simulink model "s_hover_lqrV2"  (R2012b)
settings: Solver=ode45  StartTime=0.0  StopTime=inf  FixedStep=0.01  RelTol=1e-3
values from neighbouring files (symbols this model uses):
  A = 6*(f2-f3)/z3+3*(d2+d3)    [LQRDiscretoFUNC.m]
  B = 3*(f3-f2)-z3*(d3+2*d2)    [LQRDiscretoFUNC.m]
  K = reshape(K, 4 , 6)    [LQRDiscretoFUNC.m]
undefined symbols (not defined in the file or in its folder): C, CMD_RATE_LIMIT, D, K_AMP, LQRDiscretoFUNC, V_bias, VMAX_AMP, VMAX_DAC, wcf, zetaf
libraries: simulink_extras x5, rtwinlib x1
settings Model: ExtModeTrigDuration=10000  Creator=hpineros  LastModifiedBy=David
settings SolverCC: PositivePriorityOrder=on
settings DataIOCC: SignalLoggingSaveFormat=ModelDataLogs
settings OptimizationCC: InitFltsAndDblsToZero=on
settings DebuggingCC: SaveWithParameterizedLinksMsg=none  FcnCallInpInsideContextMsg=UseLocalSettings  StrictBusMsg=Warning
settings RTWCC: SystemTargetFile=quarc_windows.tlc  TemplateMakefile=quarc_default_tmf  Description=QuaRC Win32 Target  ProcessScript=quarc_windows_make_rtw_hook
settings STFCustomTargetCC: TargetFcnLib=ansi_tfl_tmw.mat  TargetPreCompLibLocation=C:\DOCUME~1\ALLUSE~1\APPLIC~1\QUARC\lib\2007a\windows\release  CodeReplacementLibrary=ANSI_C  GeneratePreprocessorConditionals=Disable all  SystemTargetFile=quarc_windows.tlc
settings GRTTargetCC: TargetFcnLib=ansi_tfl_tmw.mat  TargetPreCompLibLocation=C:\DOCUME~1\ALLUSE~1\APPLIC~1\QUARC\lib\2007a\windows\release  ParMdlRefBuildCompliant=off  CompOptLevelCompliant=off  ConcurrentExecutionCompliant=off  CombineOutputUpdateFcns=off  MatFileLogging=off  GRTInterface=on  ExtMode=on  ExtModeMexFile=quarc_comm

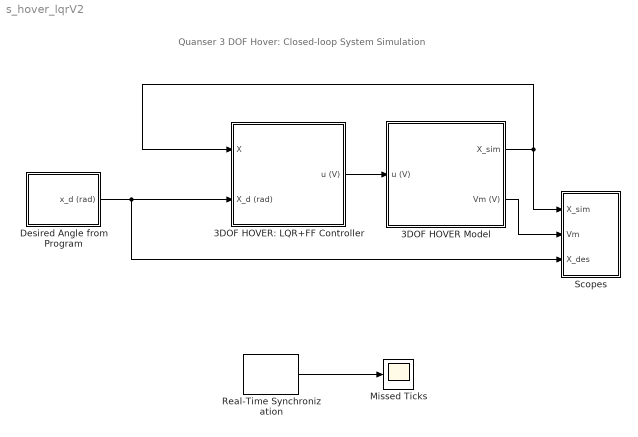
== system s_hover_lqrV2 ==
  note: Quanser 3 DOF Hover:
      | Closed-loop System Simulation
  3DOF HOVER Model : Subsystem
  3DOF HOVER: LQR+FF Controller : Subsystem
  Desired Angle from Program : Subsystem
  Missed Ticks : Scope
      settings: TickLabels=on  TimeRange=20  YMin=0  YMax=30  SaveName=ScopeData3
  Real-Time Synchronization : rtwinlib/Real-Time Synchronization  SampleTime=0.001  MaxMissedTicks=100000000000000000000000  ShowMissedTicks=on  YieldWhenWaiting=on
  Scopes : Subsystem
  wires:
  Desired Angle from Program/1(x_d (rad)) -> Scopes/3(X_des), 3DOF HOVER: LQR+FF Controller/2(X_d (rad))
  3DOF HOVER Model/1(X_sim) -> Scopes/1(X_sim), 3DOF HOVER: LQR+FF Controller/1(X)
  3DOF HOVER Model/2(Vm (V)) -> Scopes/2(Vm)
  3DOF HOVER: LQR+FF Controller/1(u (V)) -> 3DOF HOVER Model/1(u (V))
  Real-Time Synchronization/1 -> Missed Ticks/1

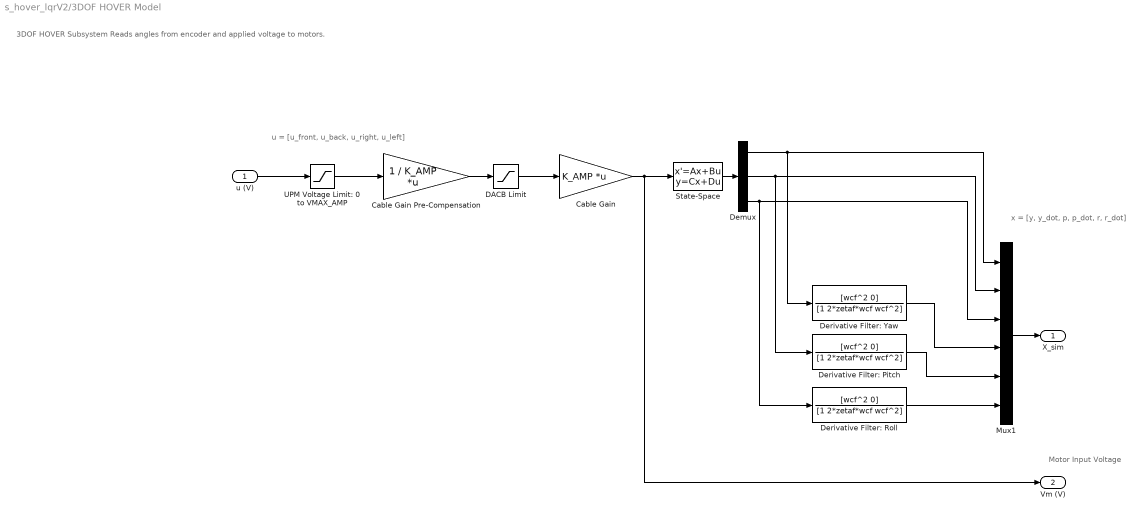
== system s_hover_lqrV2/3DOF HOVER Model ==
  note: 3DOF HOVER Subsystem
      | Reads angles from encoder and applied voltage to motors.
  note: Motor Input Voltage
  note: u = [u_front, u_back, u_right, u_left]
  note: x = [y, y_dot, p, p_dot, r, r_dot]
  u (V) : Inport
  Cable Gain : Gain  Gain=K_AMP  Multiplication=Matrix(K*u)  SaturateOnIntegerOverflow=on  OutDataTypeStr=Inherit: Same as input  ParamDataTypeStr=Inherit: Same as input
  Cable Gain Pre-Compensation : Gain  Gain=1 / K_AMP  Multiplication=Matrix(K*u)  SaturateOnIntegerOverflow=on  OutDataTypeStr=Inherit: Same as input  ParamDataTypeStr=Inherit: Same as input
  DACB Limit : Saturate  UpperLimit=VMAX_DAC  LowerLimit=-VMAX_DAC
  Demux : Demux  Outputs=3
  Derivative Filter: Pitch : TransferFcn  Numerator=[wcf^2 0]  Denominator=[1 2*zetaf*wcf wcf^2]
  Derivative Filter: Roll : TransferFcn  Numerator=[wcf^2 0]  Denominator=[1 2*zetaf*wcf wcf^2]
  Derivative Filter: Yaw : TransferFcn  Numerator=[wcf^2 0]  Denominator=[1 2*zetaf*wcf wcf^2]
  Mux1 : Mux  Inputs=6
  State-Space : StateSpace  A=A  B=B  C=C  D=D
  UPM Voltage Limit: 0 to VMAX_AMP : Saturate  UpperLimit=VMAX_AMP  LowerLimit=0
  X_sim : Outport
  Vm (V) : Outport  Port=2
  wires:
  Demux/3 -> Derivative Filter: Roll/1, Mux1/3
  Demux/2 -> Derivative Filter: Pitch/1, Mux1/2
  Derivative Filter: Roll/1 -> Mux1/6
  Derivative Filter: Pitch/1 -> Mux1/5
  Derivative Filter: Yaw/1 -> Mux1/4
  Demux/1 -> Derivative Filter: Yaw/1, Mux1/1
  State-Space/1 -> Demux/1
  Mux1/1 -> X_sim/1
  Cable Gain/1 -> State-Space/1, Vm (V)/1
  DACB Limit/1 -> Cable Gain/1
  u (V)/1 -> UPM Voltage Limit: 0 to VMAX_AMP/1
  UPM Voltage Limit: 0 to VMAX_AMP/1 -> Cable Gain Pre-Compensation/1
  Cable Gain Pre-Compensation/1 -> DACB Limit/1

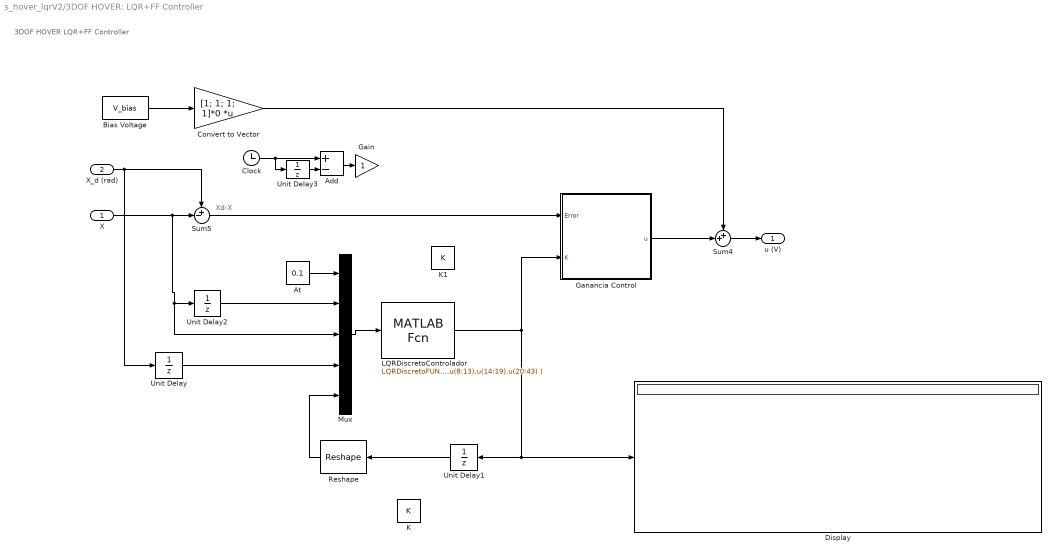
== system s_hover_lqrV2/3DOF HOVER: LQR+FF Controller ==
  note: Xd-X
  note: 3DOF HOVER LQR+FF Controller
  X : Inport
  X_d (rad) : Inport  Port=2
  Add : Sum  Inputs=+-
  At : Constant  Value=0.1
  Bias Voltage : Constant  Value=V_bias
  Clock : Clock
  Convert to Vector : Gain  Gain=[1; 1; 1; 1]*0  Multiplication=Matrix(K*u)
  Display : Display
  Gain : Gain
  Ganancia Control : MATLAB Function  TreatAsAtomicUnit=on
  K : Constant  Value=K
  K1 : Constant  Value=K
  LQRDiscretoControlador : MATLABFcn  MATLABFcn=LQRDiscretoFUNC( u(1),u(2:7),u(8:13),u(14:19),u(20:43) )  OutputDimensions=[4,6]  Output1D=off
  Mux : Mux  Inputs=5
  Reshape : Reshape  OutputDimensionality=Customize  OutputDimensions=[4*6,1]
  Sum4 : Sum  Inputs=++|
  Sum5 : Sum  Inputs=+-|
  Unit Delay : UnitDelay  InitialCondition=[0;0;0;0;0;0]  SampleTime=-1
  Unit Delay1 : UnitDelay  InitialCondition=K  SampleTime=-1
  Unit Delay2 : UnitDelay  InitialCondition=[0;0;0;0;0;0]  SampleTime=-1
  Unit Delay3 : UnitDelay  SampleTime=-1
  u (V) : Outport
  wires:
  X/1 -> Mux/3, Unit Delay2/1, Sum5/2
  X_d (rad)/1 -> Sum5/1, Unit Delay/1
  Convert to Vector/1 -> Sum4/1
  Ganancia Control/1(u) -> Sum4/2
  Bias Voltage/1 -> Convert to Vector/1
  Sum4/1 -> u (V)/1
  LQRDiscretoControlador/1 -> Display/1, Unit Delay1/1, Ganancia Control/2(K)
  Sum5/1 -> Ganancia Control/1(Error)
  Mux/1 -> LQRDiscretoControlador/1
  Unit Delay2/1 -> Mux/2
  Unit Delay/1 -> Mux/4
  Reshape/1 -> Mux/5
  Unit Delay1/1 -> Reshape/1
  Unit Delay3/1 -> Add/2
  Clock/1 -> Unit Delay3/1, Add/1
  Add/1 -> Gain/1
  At/1 -> Mux/1

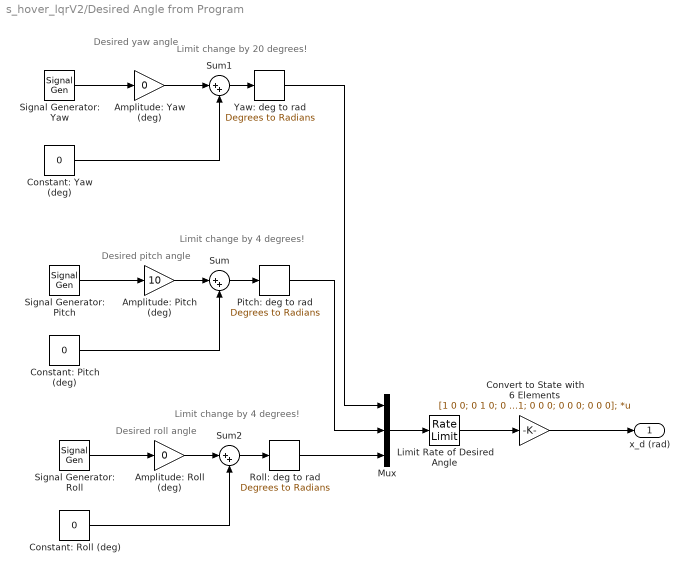
== system s_hover_lqrV2/Desired Angle from Program ==
  note: Limit change by
      | 4 degrees!
  note: Limit change by
      | 20 degrees!
  note: Limit change by
      | 4 degrees!
  note: Desired roll angle
  note: Desired pitch angle
  note: Desired yaw angle
  Amplitude: Pitch (deg) : Gain  Gain=10
  Amplitude: Roll (deg) : Gain  Gain=0
  Amplitude: Yaw (deg) : Gain  Gain=0
  Constant: Pitch (deg) : Constant  Value=0
  Constant: Roll (deg) : Constant  Value=0
  Constant: Yaw (deg) : Constant  Value=0
  Convert to State with 6 Elements : Gain  Gain=[1 0 0; 0 1 0; 0 0 1; 0 0 0; 0 0 0; 0 0 0];  Multiplication=Matrix(K*u)
  Limit Rate of Desired Angle : RateLimiter  RisingSlewLimit=CMD_RATE_LIMIT  FallingSlewLimit=-CMD_RATE_LIMIT
  Mux : Mux  Inputs=3
  Pitch: deg to rad : simulink_extras/Transformations/Degrees to Radians
  Roll: deg to rad : simulink_extras/Transformations/Degrees to Radians
  Signal Generator: Pitch : SignalGenerator  WaveForm=square  Frequency=0.1
  Signal Generator: Roll : SignalGenerator  WaveForm=square  Frequency=0.08
  Signal Generator: Yaw : SignalGenerator  WaveForm=square  Frequency=0.4
  Sum : Sum  Inputs=|++
  Sum1 : Sum  Inputs=|++
  Sum2 : Sum  Inputs=|++
  Yaw: deg to rad : simulink_extras/Transformations/Degrees to Radians
  x_d (rad) : Outport
  wires:
  Convert to State with 6 Elements/1 -> x_d (rad)/1
  Limit Rate of Desired Angle/1 -> Convert to State with 6 Elements/1
  Roll: deg to rad/1 -> Mux/3
  Pitch: deg to rad/1 -> Mux/2
  Yaw: deg to rad/1 -> Mux/1
  Sum2/1 -> Roll: deg to rad/1
  Signal Generator: Roll/1 -> Amplitude: Roll (deg)/1
  Amplitude: Roll (deg)/1 -> Sum2/1
  Constant: Roll (deg)/1 -> Sum2/2
  Sum/1 -> Pitch: deg to rad/1
  Signal Generator: Pitch/1 -> Amplitude: Pitch (deg)/1
  Amplitude: Pitch (deg)/1 -> Sum/1
  Constant: Pitch (deg)/1 -> Sum/2
  Sum1/1 -> Yaw: deg to rad/1
  Signal Generator: Yaw/1 -> Amplitude: Yaw (deg)/1
  Amplitude: Yaw (deg)/1 -> Sum1/1
  Constant: Yaw (deg)/1 -> Sum1/2
  Mux/1 -> Limit Rate of Desired Angle/1

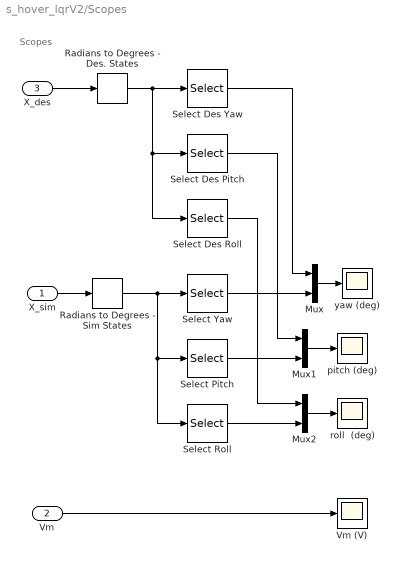
== system s_hover_lqrV2/Scopes ==
  note: Scopes
  X_sim : Inport
  Vm : Inport  Port=2
  X_des : Inport  Port=3
  Mux : Mux  Inputs=2
  Mux1 : Mux  Inputs=2
  Mux2 : Mux  Inputs=2
  Radians to Degrees - Des. States : simulink_extras/Transformations/Radians to Degrees
  Radians to Degrees - Sim States : simulink_extras/Transformations/Radians to Degrees
  Select Des Pitch : Selector  InputPortWidth=6  IndexOptions=Index vector (dialog)  Indices=2  OutputSizes=1
  Select Des Roll : Selector  InputPortWidth=6  IndexOptions=Index vector (dialog)  Indices=3  OutputSizes=1
  Select Des Yaw : Selector  InputPortWidth=6  IndexOptions=Index vector (dialog)  Indices=1  OutputSizes=1
  Select Pitch : Selector  InputPortWidth=6  IndexOptions=Index vector (dialog)  Indices=2  OutputSizes=1
  Select Roll : Selector  InputPortWidth=6  IndexOptions=Index vector (dialog)  Indices=3  OutputSizes=1
  Select Yaw : Selector  InputPortWidth=6  IndexOptions=Index vector (dialog)  Indices=1  OutputSizes=1
  Vm (V) : Scope
      settings: TickLabels=on  TimeRange=20  YMin=-15  YMax=15  SaveName=ScopeData4
  pitch (deg) : Scope
      settings: TickLabels=on  TimeRange=20  YMin=-11  YMax=11
  roll  (deg) : Scope
      settings: TickLabels=on  TimeRange=20  SaveName=ScopeData2
  yaw (deg) : Scope
      settings: TickLabels=on  TimeRange=20  YMin=-0.9  YMax=0.1
  wires:
  Select Des Roll/1 -> Mux2/1
  Select Des Pitch/1 -> Mux1/1
  Select Des Yaw/1 -> Mux/1
  Radians to Degrees - Des. States/1 -> Select Des Roll/1, Select Des Pitch/1, Select Des Yaw/1
  Select Roll/1 -> Mux2/2
  Select Pitch/1 -> Mux1/2
  Select Yaw/1 -> Mux/2
  Mux2/1 -> roll  (deg)/1
  Radians to Degrees - Sim States/1 -> Select Roll/1, Select Pitch/1, Select Yaw/1
  Vm/1 -> Vm (V)/1
  Mux1/1 -> pitch (deg)/1
  Mux/1 -> yaw (deg)/1
  X_sim/1 -> Radians to Degrees - Sim States/1
  X_des/1 -> Radians to Degrees - Des. States/1

== matlab function s_hover_lqrV2/3DOF HOVER: LQR+FF Controller/Ganancia Control ==
  data: u output; Error input; K input
function u = GananciaLQR(Error,K)

u=K*Error;
